simulink library "csc_ltg_landing_terminal_guidance_mtv_lib"  (R2014b)
settings: Solver=ode45  StartTime=0.0  StopTime=10.0  RelTol=1e-3
undefined symbols (not defined in the file or in its folder): fsw_dt, kd_lateral, ki_lateral, kp_lateral, lateral_control_angle_max
libraries: util_common_lib x3, simulink x2, util_info_lib x1, csc_tlt_takeoff_landing_table_guidance_mtv_lib x1, util_extra_lib x1
settings Model: Creator=escrane  LastModifiedBy=tgorton

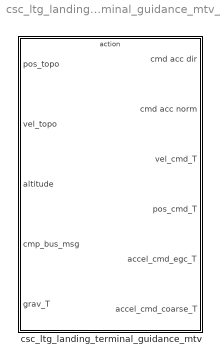
== system csc_ltg_landing_terminal_guidance_mtv_lib ==
  csc_ltg_landing_terminal_guidance_mtv : Subsystem  TreatAsAtomicUnit=on

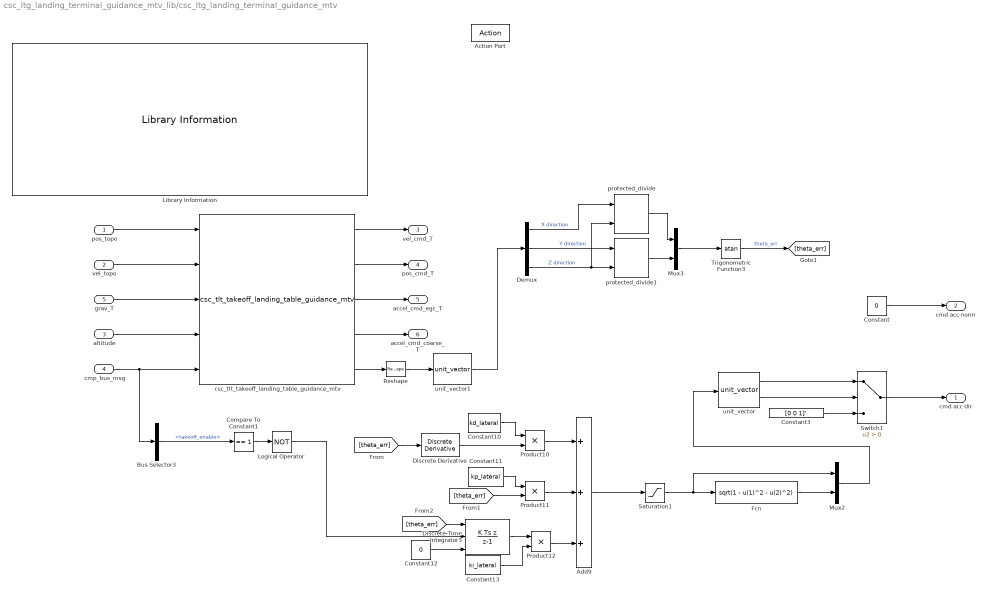
== system csc_ltg_landing_terminal_guidance_mtv_lib/csc_ltg_landing_terminal_guidance_mtv ==
  pos_topo : Inport
  vel_topo : Inport  Port=2
  altitude : Inport  Port=3
  cmp_bus_msg : Inport  Port=4
  grav_T : Inport  Port=5
  Action Port : ActionPort
  Add9 : Sum  Inputs=+++
  Bus Selector3 : BusSelector  OutputSignals=takeoff_enable
  Compare To Constant1 : simulink/Logic and Bit Operations/Compare To Constant  relop===  const=1  OutDataTypeStr=boolean
  Constant : Constant  Value=0
  Constant10 : Constant  Value=kd_lateral
  Constant11 : Constant  Value=kp_lateral
  Constant12 : Constant  Value=0
  Constant13 : Constant  Value=ki_lateral
  Constant3 : Constant  Value=[0 0 1]'
  Demux : Demux  Outputs=3
  Discrete Derivative : simulink/Discrete/Discrete Derivative  gainval=1.0  ICPrevScaledInput=0.0  InputProcessing=Inherited  OutMin=[]  OutMax=[]  OutDataType=fixdt(1, 16)  OutScaling=2^-10  DoSatur=off
  Discrete-Time Integrator3 : DiscreteIntegrator  IntegratorMethod=Integration: Backward Euler  gainval=1  ExternalReset=level  InitialConditionSource=external  InitialConditionSetting=State (most efficient)  SampleTime=fsw_dt  LimitOutput=on  UpperSaturationLimit=1e6  LowerSaturationLimit=-1e6
  Fcn : Fcn  Expr=sqrt(1 - u(1)^2 - u(2)^2)
  Library Information : util_info_lib/Library Information  owner='NONE'
  Logical Operator : Logic  Operator=NOT  AllPortsSameDT=off  OutDataTypeStr=boolean
  Mux2 : Mux  Inputs=[2 1]
  Mux3 : Mux  Inputs=2
  Product10 : Product
  Product11 : Product
  Product12 : Product
  Reshape : Reshape
  Saturation1 : Saturate  UpperLimit=lateral_control_angle_max  LowerLimit=-lateral_control_angle_max
      settings: AttributesFormatString=|
      | %<UpperLimit>
      | %<LowerLimit>
  Switch1 : Switch  Criteria=u2 > Threshold
  Trigonometric Function3 : Trigonometry  Operator=atan
  csc_tlt_takeoff_landing_table_guidance_mtv : csc_tlt_takeoff_landing_table_guidance_mtv_lib/csc_tlt_takeoff_landing_table_guidance_mtv  VariantControl=tlt_altitude_takeoff_table
  protected_divide : util_common_lib/protected_divide  fault_value=0  tolerance=eps
  protected_divide1 : util_common_lib/protected_divide  fault_value=0  tolerance=eps
  unit_vector : util_extra_lib/unit_vector  SystemSampleTime=-1
  unit_vector1 : util_common_lib/unit_vector  SystemSampleTime=-1
  cmd acc dir : Outport
  cmd acc norm : Outport  Port=2
  vel_cmd_T : Outport  Port=3  InitialOutput=0
  pos_cmd_T : Outport  Port=4  InitialOutput=0
  accel_cmd_egc_T : Outport  Port=5
  accel_cmd_coarse_T : Outport  Port=6
  wires:
  protected_divide1/1 -> Mux3/2
  Mux3/1 -> Trigonometric Function3/1
  protected_divide/1 -> Mux3/1
  Reshape/1 -> unit_vector1/1
  Mux2/1 -> unit_vector/1
  Saturation1/1 -> Fcn/1, Mux2/1
  Trigonometric Function3/1 -> [theta_err]  "theta_err"
  Fcn/1 -> Mux2/2
  Demux/3 -> protected_divide/2, protected_divide1/2  "Z direction"
  Demux/2 -> protected_divide1/1  "Y direction"
  Demux/1 -> protected_divide/1  "X direction"
  Add9/1 -> Saturation1/1
  Discrete Derivative/1 -> Product10/2
  Logical Operator/1 -> Discrete-Time Integrator3/2
  Compare To Constant1/1 -> Logical Operator/1
  Bus Selector3/1 -> Compare To Constant1/1  "<takeoff_enable>"
  Product12/1 -> Add9/3
  Discrete-Time Integrator3/1 -> Product12/1
  Constant13/1 -> Product12/2
  Constant12/1 -> Discrete-Time Integrator3/3
  [theta_err] -> Discrete-Time Integrator3/1
  Product11/1 -> Add9/2
  Product10/1 -> Add9/1
  Constant11/1 -> Product11/1
  Constant10/1 -> Product10/1
  [theta_err] -> Product11/2
  [theta_err] -> Discrete Derivative/1
  csc_tlt_takeoff_landing_table_guidance_mtv/5 -> Reshape/1
  unit_vector1/1 -> Demux/1
  csc_tlt_takeoff_landing_table_guidance_mtv/3 -> accel_cmd_egc_T/1
  csc_tlt_takeoff_landing_table_guidance_mtv/4 -> accel_cmd_coarse_T/1
  unit_vector/1 -> Switch1/1
  Constant3/1 -> Switch1/3
  unit_vector/2 -> Switch1/2
  Switch1/1 -> cmd acc dir/1
  csc_tlt_takeoff_landing_table_guidance_mtv/2 -> pos_cmd_T/1
  csc_tlt_takeoff_landing_table_guidance_mtv/1 -> vel_cmd_T/1
  Constant/1 -> cmd acc norm/1
  altitude/1 -> csc_tlt_takeoff_landing_table_guidance_mtv/4
  vel_topo/1 -> csc_tlt_takeoff_landing_table_guidance_mtv/2
  pos_topo/1 -> csc_tlt_takeoff_landing_table_guidance_mtv/1
  grav_T/1 -> csc_tlt_takeoff_landing_table_guidance_mtv/3
  cmp_bus_msg/1 -> Bus Selector3/1, csc_tlt_takeoff_landing_table_guidance_mtv/5
